simulink model "CMPE243_MPT1_Group-2_Şimal_Ersuz_Overall _K-MAP_System"  (R2025a)
settings: Solver=VariableStepAuto  StartTime=0.0  StopTime=10.0  RelTol=1e-3
settings Model: Creator=simalersuz  LastModifiedBy=simalersuz

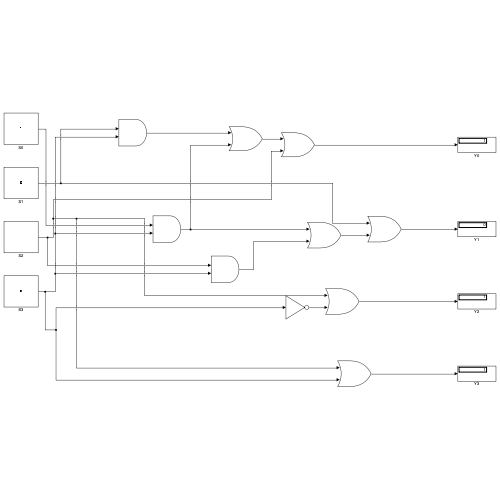
[thumbnail: Simulink's stored preview of the top-level diagram]
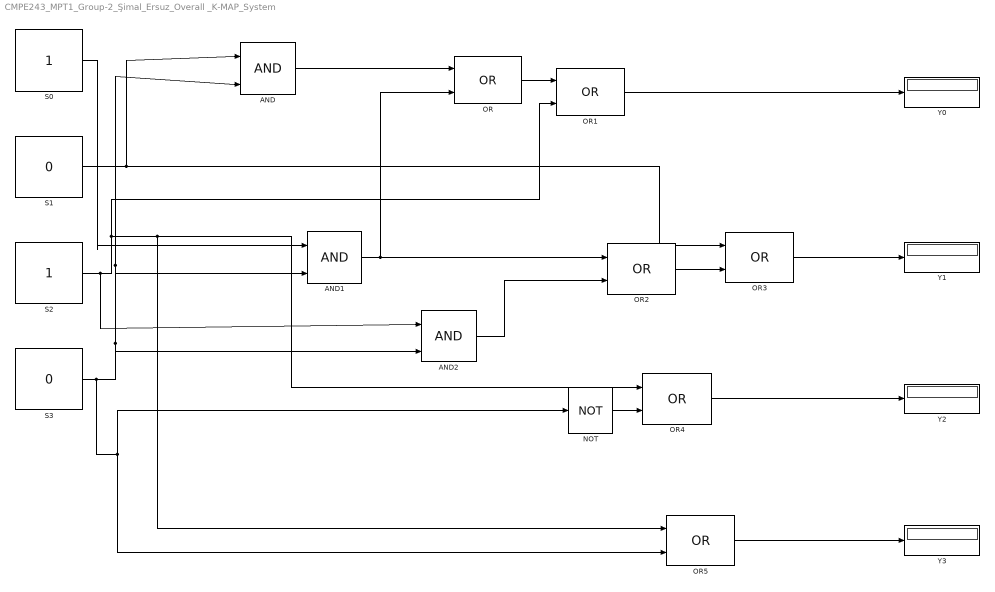
== system CMPE243_MPT1_Group-2_Şimal_Ersuz_Overall _K-MAP_System ==
  AND : Logic  IconShape=distinctive  AllPortsSameDT=off  OutDataTypeStr=boolean
  AND1 : Logic  IconShape=distinctive  AllPortsSameDT=off  OutDataTypeStr=boolean
  AND2 : Logic  IconShape=distinctive  AllPortsSameDT=off  OutDataTypeStr=boolean
  NOT : Logic  Operator=NOT  IconShape=distinctive  AllPortsSameDT=off  OutDataTypeStr=boolean
  OR{,1..5} (6 alike) : Logic  Operator=OR  IconShape=distinctive  AllPortsSameDT=off  OutDataTypeStr=boolean
  S0 : Constant
  S1 : Constant  Value=0
  S2 : Constant
  S3 : Constant  Value=0
  Y{0..3} (4 alike) : Display
  wires:
  S3/1 -> OR5/2, NOT/1, AND1/2, AND/2, AND2/2
  S1/1 -> AND/1, OR3/1
  S0/1 -> AND1/1
  AND/1 -> OR/1
  AND1/1 -> OR/2, OR2/1
  S2/1 -> AND2/1, OR1/2, OR5/1, OR4/1
  OR/1 -> OR1/1
  AND2/1 -> OR2/2
  OR2/1 -> OR3/2
  NOT/1 -> OR4/2
  OR5/1 -> Y3/1
  OR4/1 -> Y2/1
  OR3/1 -> Y1/1
  OR1/1 -> Y0/1
